simulink model "mov_rot_sim"  (R2022b)
settings: Solver=VariableStepAuto  StartTime=0.0  StopTime=10.0  MaxStep=0.001  RelTol=1e-3
values from neighbouring files (symbols this model uses):
  k = 100    [MOV_ROT.m]    (also in datos_simulink.m)
  m = 10    [MOV_ROT.m]    (also in datos_simulink.m)
  r = 0.05    [MOV_ROT.m]    (also in datos_simulink.m)
libraries: fl_lib x5, nesl_utility x3
settings Model: Creator=Cris  LastModifiedBy=Cris

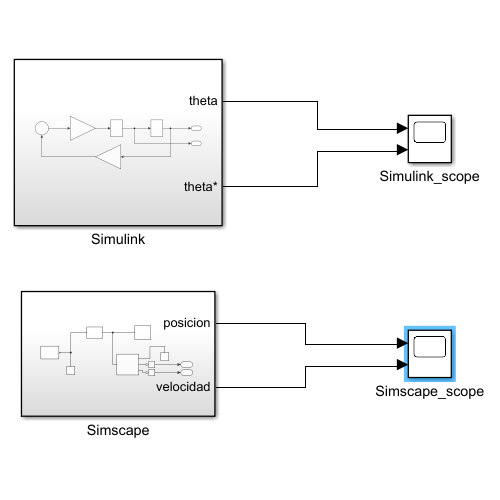
[thumbnail: Simulink's stored preview of the top-level diagram]
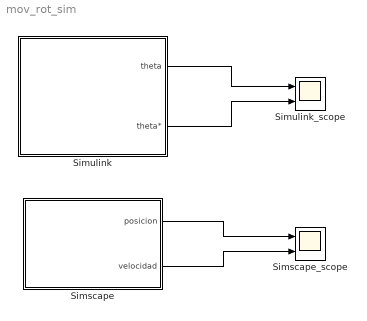
== system mov_rot_sim ==
  Simscape : Subsystem
  Simscape_scope : Scope  NumInputPorts=2
  Simulink : Subsystem
  Simulink_scope : Scope  NumInputPorts=2
  wires:
  Simulink/1(theta) -> Simulink_scope/1
  Simulink/2(theta*) -> Simulink_scope/2
  Simscape/1(posicion) -> Simscape_scope/1
  Simscape/2(velocidad) -> Simscape_scope/2

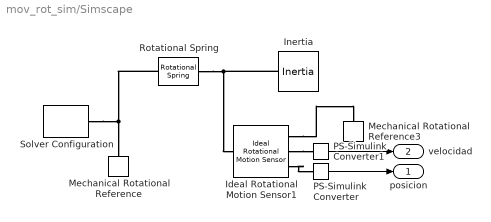
== system mov_rot_sim/Simscape ==
  Ideal Rotational Motion Sensor1 : fl_lib/Mechanical/Mechanical Sensors/Ideal Rotational Motion Sensor  reference=foundation.enum.MeasurementReference.difference  acceleration_port=false  velocity_port=true  position_port=true  wrap_angle=false  offset=20 deg
  Inertia : fl_lib/Mechanical/Rotational Elements/Inertia  inertia=3*(m*r^2)/2 kg*m^2  num_ports=foundation.enum.numPorts2.one  w_specify=off  w_priority=High  w=0 rad/s  w_nominal_specify=off  w_nominal_unit=rad/s  w_nominal_value=1  t_specify=off  t_priority=None  t=0 N*m  t_nominal_specify=off  t_nominal_unit=N*m  t_nominal_value=1
  Mechanical Rotational Reference : fl_lib/Mechanical/Rotational Elements/Mechanical Rotational Reference
  Mechanical Rotational Reference3 : fl_lib/Mechanical/Rotational Elements/Mechanical Rotational Reference
  PS-Simulink Converter : nesl_utility/PS-Simulink Converter  PhysicalDomain=network_engine_domain  SubClassName=ps_output  LeftPortType=input  RightPortType=output  PseudoPeriodic=off  Frequencies=[]  VectorFormat=inherit  Unit=inherit  AffineConversion=off
  PS-Simulink Converter1 : nesl_utility/PS-Simulink Converter  PhysicalDomain=network_engine_domain  SubClassName=ps_output  LeftPortType=input  RightPortType=output  PseudoPeriodic=off  Frequencies=[]  VectorFormat=inherit  Unit=inherit  AffineConversion=off
  Rotational Spring : fl_lib/Mechanical/Rotational Elements/Rotational Spring  spr_rate=k*r N*m/rad  w_specify=off  w_priority=High  w=0 rad/s  w_nominal_specify=off  w_nominal_unit=rad/s  w_nominal_value=1  t_specify=off  t_priority=High  t=k N*m  t_nominal_specify=off  t_nominal_unit=N*m  t_nominal_value=k  phi_specify=on  phi_priority=High  phi=20*pi/180 rad  phi_nominal_specify=off  phi_nominal_unit=rad  phi_nominal_value=1
  Solver Configuration : nesl_utility/Solver Configuration  PhysicalDomain=network_engine_domain  SubClassName=solver  LeftPortType=input  RightPortType=generic  Tones=[]  Harmonics=[]  SimulateNoise=off  Profile=off  UseLocalSampling=off  EnableSwitchedLinearOptims=on  FrequencyDomain=off  UseCCode=off  RelTol=0.001  AbsTol=0.001  MinStep=1e-09  ToWorkspace=off  RevertToSquareIcSolve=off  NumHomotopyIterations=100  PhasorMode=off  PhasorModeNumHarmonics=1  ConsistencySolver=NEWTON_XTOL_AFTER_FTOL  IndexReductionMethod=DerivativeReplacement  DoDC=off  ResidualTolerance=1e-09  ConsistencyTolSource=GLOBAL  ConsistencyAbsTol=0.001  ConsistencyRelTol=0.001  ConsistencyTolFactor=0.001  UseLocalSolver=off  LocalSolverChoice=NE_BACKWARD_EULER_ADVANCER  ResolveIndetEquations=on  FunctionEvalNumThread=1  LocalSolverSampleTime=0.001  DoFixedCost=off  MaxNonlinIter=3  MaxModeIter=2  ComputeImpulses=off  ImpulseIterations=2  LinearAlgebra=auto  LinearAlgebraNumThread=0  EquationFormulation=NE_TIME_EF  DelaysMemoryBudget=1024  AutomaticFiltering=on  FilteringTimeConstant=0.001  PartitionStorageMethod=AS_NEEDED  PartitionMemoryBudget=1024  PartitionMethod=ROBUST
  posicion : Outport
  velocidad : Outport  Port=2
  wires:
  PS-Simulink Converter/1 -> posicion/1
  PS-Simulink Converter1/1 -> velocidad/1
  connections:
  Ideal Rotational Motion Sensor1/RConn1 -- Mechanical Rotational Reference3/LConn1
  Solver Configuration/RConn1 -- Mechanical Rotational Reference/LConn1 -- Rotational Spring/RConn1
  Inertia/LConn1 -- Rotational Spring/LConn1 -- Ideal Rotational Motion Sensor1/LConn1
  Ideal Rotational Motion Sensor1/RConn2 -- PS-Simulink Converter1/LConn1
  Ideal Rotational Motion Sensor1/RConn3 -- PS-Simulink Converter/LConn1

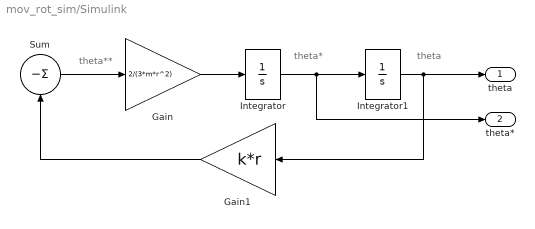
== system mov_rot_sim/Simulink ==
  note: theta**
  note: theta*
  note: theta
  Gain : Gain  Gain=2/(3*m*r^2)
  Gain1 : Gain  Gain=k*r
  Integrator : Integrator
  Integrator1 : Integrator  InitialCondition=20*pi/180
  Sum : Sum  Inputs=|-
  theta : Outport
  theta* : Outport  Port=2
  wires:
  Sum/1 -> Gain/1
  Gain1/1 -> Sum/1
  Integrator/1 -> theta*/1, Integrator1/1
  Integrator1/1 -> theta/1, Gain1/1
  Gain/1 -> Integrator/1
